simulink model "stateflow_unconditionflow"  (R2016b)
settings: Solver=VariableStepAuto  StartTime=0.0  StopTime=10.0  RelTol=1e-3  EnableMultiTasking=on
settings Model: Creator=amyyang  LastModifiedBy=amyyang
settings DataIOCC: LimitDataPoints=on
settings OptimizationCC: LifeSpan=inf
settings DebuggingCC: AllowSymbolicDim=off  SFUnexpectedBacktrackingDiag=warning  SFNoUnconditionalDefaultTransitionDiag=warning  SFExecutionAtInitializationDiag=none
settings ModelReferenceCC: PropagateSignalLabelsOutOfModel=off
settings GRTTargetCC: TargetLangStandard=C89/C90 (ANSI)
settings ConfigComp: CovMetricSettings=dw  CovHtmlReporting=on  CovSaveCumulativeToWorkspaceVar=on  CovSaveSingleToWorkspaceVar=on  CovExternalEMLEnable=off

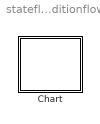
== system stateflow_unconditionflow ==
  Chart : Stateflow chart  TreatAsAtomicUnit=on

== stateflow chart stateflow_unconditionflow/Chart ==
  note: 所以，为了避免误解，需要
      | 复杂条件不要用Junction分开单独写；
      | 提供无条件路径
  state B [parallel]
    settings: executionOrder=2
    note: 当 C1 == ON， 而 C2 == OFF时，
        | 熟悉的工程师可以推理得出 out =0，
        | 但是为了避免误解，需要避免这种写法。
    (default) -> (junction 135)
    (junction 135) -> (junction 137) [order 1] : [ C1 == ON]
    (junction 137) -> (junction 133) : [C2 == ON]
    (junction 135) -> (junction 130) [order 2] : {
        |  out = 0;
        | }
    (junction 133) -> (junction 132) : {
        |  out = 1;
        | }
    (junction 132) -> (junction 130)
    (junction 130) -> (junction 134)
  state A [parallel]
    settings: executionOrder=1
    note: 防止Backtracking
    (default) -> (junction 114)
    (junction 114) -> (junction 115) [order 1] : [ (C1 == ON) && (C2 == ON)]
    (junction 114) -> (junction 116) [order 2] : {
        |  out = 0;
        | }
    (junction 115) -> (junction 117) : {
        |  out = 1;
        | }
    (junction 117) -> (junction 116)
    (junction 116) -> (junction 122)
